simulink model "Model"  (R2013b)
settings: Solver=ode4  StartTime=0.0  StopTime=10.0  FixedStep=1e-3  RelTol=1e-3
values from neighbouring files (symbols this model uses):
  D = xopt(3)    [Plant1delay.m]    (also in Plant2.m; Plant2delay.m; Plant3.m; Plant4.m)
  I = xopt(2)    [Plant1delay.m]    (also in Plant2.m; Plant2delay.m; Plant3.m; Plant4.m)
  N = xopt(4)    [Plant1delay.m]    (also in Plant2.m; Plant2delay.m; Plant3.m; Plant4.m)
  P = xopt(1)    [Plant1delay.m]    (also in Plant2.m; Plant2delay.m; Plant3.m; Plant4.m)
undefined symbols (not defined in the file or in its folder): kG, pG
libraries: simulink_extras x1
settings Model: Creator=stelmo  LastModifiedBy=stelmo

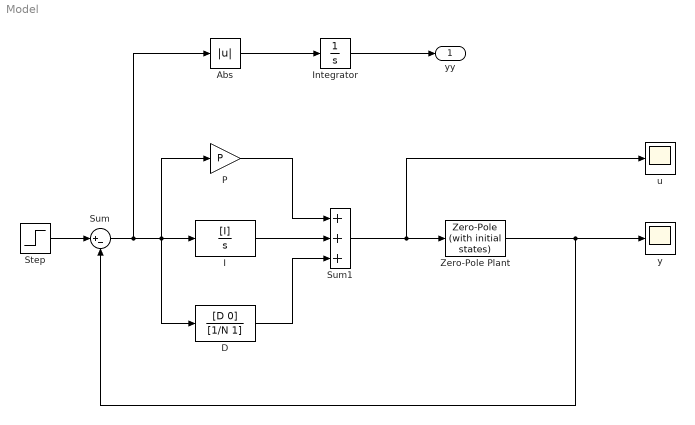
== system Model ==
  Abs : Abs
  D : TransferFcn  Numerator=[D 0]  Denominator=[1/N 1]
  I : TransferFcn  Numerator=[I]  Denominator=[1 0]
  Integrator : Integrator
  P : Gain  Gain=P
  Step : Step  SampleTime=0
  Sum : Sum  Inputs=|+-
  Sum1 : Sum  Inputs=+++
  Zero-Pole Plant : simulink_extras/Additional Linear/Zero-Pole (with initial states)  Z=zG  P=pG  K=kG  X0=0
  u : Scope
  y : Scope
  yy : Outport
  wires:
  Step/1 -> Sum/1
  Sum/1 -> Abs/1, D/1, P/1, I/1
  P/1 -> Sum1/1
  I/1 -> Sum1/2
  D/1 -> Sum1/3
  Zero-Pole Plant/1 -> y/1, Sum/2
  Abs/1 -> Integrator/1
  Integrator/1 -> yy/1
  Sum1/1 -> u/1, Zero-Pole Plant/1
